simulink model "FAST_EMPC"  (R2021a)
settings: Solver=ode4  StartTime=0.0  StopTime=TMax  FixedStep=DT  MaxStep=DT  RelTol=1e-3  EnableMultiTasking=on
values from neighbouring files (symbols this model uses):
  Drivetrain =     [NREL5MW.mat]
  luenGainDisc = place(sys_tower_fa_d_obsv.A',sys_tower_fa_d_obsv.C',luenPolesDisc)'    [Init_FAST_EMPC.m]
  Parameters =     [Parameters.mat]
  RPM_Init = 9.4965    [Init_FAST_EMPC.m]
  sys_tower_fa_d_obsv = c2d(sys_tower_ss_obsv,Parameters.TsObsv,'tustin')    [Init_FAST_EMPC.m]
  sys_tower_fa_d_obsv_mode = c2d(sys_tower_ss_obsv_mode,Parameters.TsObsv,'tustin')    [Init_FAST_EMPC.m]
undefined symbols (not defined in the file or in its folder): EMPCController_Tower, luenGainDisc2, luenGainDisc_comp, OutList, strmatch, sys_tower_fa_d_obsv2, sys_tower_fa_d_obsv_comp
libraries: dspstat3 x8
(part 2 of 2)

== matlab function FAST_EMPC/EMPC/Pav Coefficients/Constraints_PW1 ==
  settings: updateMethod=DISCRETE  sampleTime=Parameters.TsMPC
  data: currentV input size=1; AA output size=[Parameters.Nconst 1]; BB output size=[Parameters.Nconst 1]; Parameters parameter
function [AA,BB]  = fcn(currentV, Parameters)
currentV=max(min(currentV,25),2);

AA=zeros(Parameters.Nconst,1);
BB=zeros(Parameters.Nconst,1);

[~,qq]=max(((Parameters.BOUNDPW.V-currentV)>=0)*-50+Parameters.BOUNDPW.V-currentV);
fraction=1-(currentV-Parameters.BOUNDPW.V(qq))/(Parameters.BOUNDPW.V(qq+1)-Parameters.BOUNDPW.V(qq));

AA=(Parameters.BOUNDPW.Ac(:,qq)*fraction+Parameters.BOUNDPW.Ac(:,qq+1)*(1-fraction));
BB=(Parameters.BOUNDPW.Bc(:,qq)*fraction+Parameters.BOUNDPW.Bc(:,qq+1)*(1-fraction));

== matlab function FAST_EMPC/MATLAB Function3 ==
  data: ASensor1 input; ASensor2 input; Amode2 output; Parameters parameter
function Amode2  = fcn(ASensor1,ASensor2,Parameters)

Amode2 = -(Parameters.StaticPosition2(1)*ASensor1 - Parameters.StaticPosition1(1) * ASensor2)...
         /(Parameters.StaticPosition1(1)*Parameters.StaticPosition2(2)-Parameters.StaticPosition2(1)*Parameters.StaticPosition1(2));

== matlab function FAST_EMPC/EMPC/omega_g to K ==
  data: u input; K output; Parameters parameter
function K = calc_kin_en(u, Parameters)

K = 1/2*Parameters.Je*u^2;

== matlab function FAST_EMPC/InputInterpolator/MATLAB Function1 ==
  settings: updateMethod=CONTINUOUS  sampleTime=0.1
  data: u input size=1; y output size=1; t input; Parameters parameter
function y  = fcn(u,t,Parameters)
persistent u1 u2

% 1) Initialize
if isempty(u1)
    u1 = 1;
    u2 = 0;
end

% 2) Check if u has changed
tt = mod(t,Parameters.TsMPC);
if tt == 0
    % if so, assign u2 to u1
    u1 = u2;
    % and u to u2
    u2 = u;
end

% 3) Calculate output
y = (u2-u1)/Parameters.TsMPC*tt+u1;

== matlab function FAST_EMPC/InputInterpolator/MATLAB Function2 ==
  settings: updateMethod=CONTINUOUS  sampleTime=0.1
  data: u input size=1; y output size=1; t input; Parameters parameter
function y  = fcn(u,t,Parameters)
persistent u1 u2

% 1) Initialize
if isempty(u1)
    u1 = 0;
    u2 = 0;
end

% 2) Check if u has changed
tt = mod(t,Parameters.TsMPC);
if tt == 0
    % if so, assign u2 to u1
    u1 = u2;
    % and u to u2
    u2 = u;
end

% 3) Calculate output
y = (u2-u1)/Parameters.TsMPC*tt+u1;

== matlab function FAST_EMPC/MATLAB Function2 ==
  data: ASensor1 input; ASensor2 input; Amode1 output; Parameters parameter
function Amode1  = fcn(ASensor1,ASensor2,Parameters)

Amode1 = (Parameters.StaticPosition2(2)*ASensor1 - Parameters.StaticPosition1(2) * ASensor2)...
         /(Parameters.StaticPosition1(1)*Parameters.StaticPosition2(2)-Parameters.StaticPosition2(1)*Parameters.StaticPosition1(2));

== matlab function FAST_EMPC/Subsystem2/MATLAB Function ==
  data: v input; FT output; pitch input; omega_r_in input; Parameters parameter
function FT = fcn(v,pitch,omega_r_in,Parameters)

omega_r = omega_r_in *pi/30;
TSR = omega_r*Parameters.R/v;

ct = interp2(Parameters.Rotor_Lamda,Parameters.Rotor_PitchFull,Parameters.Rotor_cTFull,TSR,pitch,'spline');

FT = 1/2*Parameters.rho*pi*Parameters.R^2*ct*v^2;

== matlab function FAST_EMPC/EMPC/Subsystem/DeriveK ==
  settings: updateMethod=DISCRETE  sampleTime=Ts
  data: omega_g input; K output; Parameters parameter
function K = fcn(omega_g, Parameters)

K = 1/2*Parameters.J*omega_g^2;

== matlab function FAST_EMPC/InputInterpolator/MATLAB Function5 ==
  settings: updateMethod=CONTINUOUS  sampleTime=0.1
  data: u input size=1; y output size=1; t input; Parameters parameter
function y  = fcn(u,t,Parameters)
persistent u1 u2

% 1) Initialize
if isempty(u1)
    u1 = 0;
    u2 = 0;
end

% 2) Check if u has changed
tt = mod(t,Parameters.TsMPC);
if tt == 0
    % if so, assign u2 to u1
    u1 = u2;
    % and u to u2
    u2 = u;
end

% 3) Calculate output
y = (u2-u1)/Parameters.TsMPC*tt+u1;

== matlab function FAST_EMPC/Subsystem/MATLAB Function ==
  data: v input; FT output; pitch input; omega_r_in input; Parameters parameter
function FT = fcn(v,pitch,omega_r_in,Parameters)

omega_r = omega_r_in *pi/30;
TSR = omega_r*Parameters.R/v;

ct = interp2(Parameters.Rotor_Lamda,Parameters.Rotor_PitchFull,Parameters.Rotor_cTFull,TSR,pitch,'spline');

FT = 1/2*Parameters.rho*pi*Parameters.R^2*ct*v^2;

== matlab function FAST_EMPC/Subsystem1/MATLAB Function ==
  data: v input; FT output; pitch input; omega_r_in input; Parameters parameter
function FT = fcn(v,pitch,omega_r_in,Parameters)

omega_r = omega_r_in *pi/30;
TSR = omega_r*Parameters.R/v;

ct = interp2(Parameters.Rotor_Lamda,Parameters.Rotor_PitchFull,Parameters.Rotor_cTFull,TSR,pitch,'spline');

FT = 1.25*1/2*Parameters.rho*pi*Parameters.R^2*ct*v^2;
